simulink model "sampleModel1873_5_sub_sub"  (R2023a)
settings: Solver=VariableStepAuto  StartTime=0.0  StopTime=10.0  RelTol=1e-3
libraries: hdlsllib x7, simulink x1
settings Model: Creator=user1  LastModifiedBy=user1

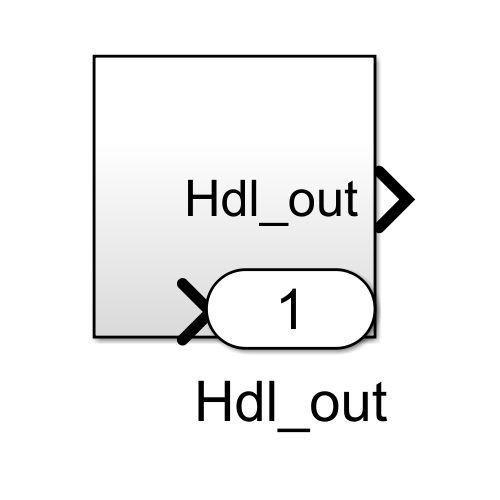
[thumbnail: Simulink's stored preview of the top-level diagram]
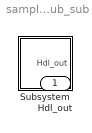
== system sampleModel1873_5_sub_sub ==
  Subsystem : Subsystem
  Hdl_out : Outport  OutDataTypeStr=uint8

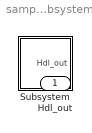
== system sampleModel1873_5_sub_sub/Subsystem ==
  Subsystem : Subsystem
  Hdl_out : Outport  OutDataTypeStr=uint8

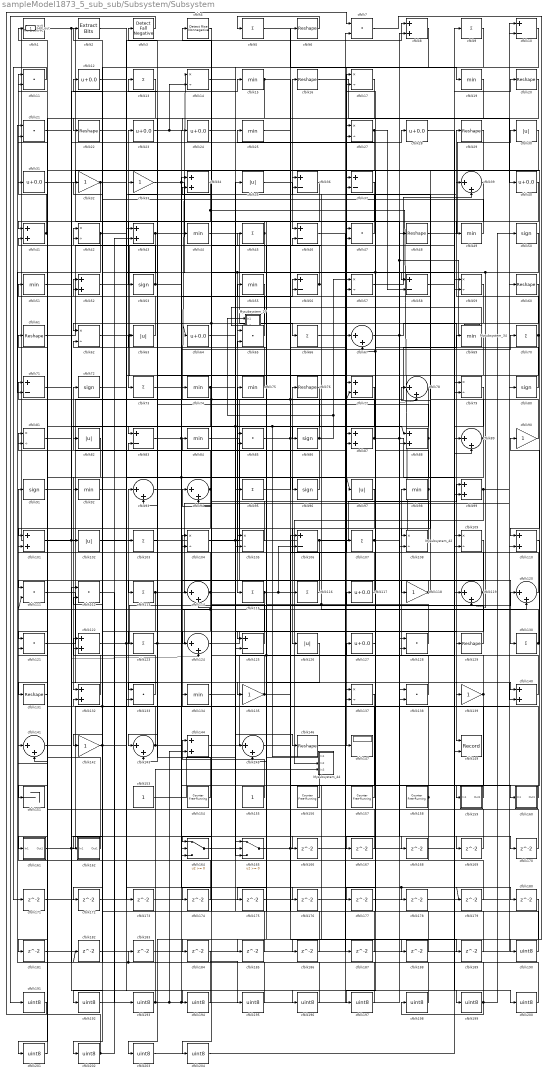
== system sampleModel1873_5_sub_sub/Subsystem/Subsystem ==
  Mysubsystem_27 : Subsystem  TreatAsAtomicUnit=on  RTWFcnName=Mysubsystem_27
      settings: RTWFcnNameOpts=User specified  RTWFileNameOpts=Use function name
  Mysubsystem_34 : Subsystem  TreatAsAtomicUnit=on  RTWFcnName=Mysubsystem_34
      settings: RTWFcnNameOpts=User specified  RTWFileNameOpts=Use function name
  Mysubsystem_42 : Subsystem  TreatAsAtomicUnit=on  RTWFcnName=Mysubsystem_42
      settings: RTWFcnNameOpts=User specified  RTWFileNameOpts=Use function name
  Mysubsystem_44 : Subsystem  TreatAsAtomicUnit=on  RTWFcnName=Mysubsystem_44
      settings: RTWFcnNameOpts=User specified  RTWFileNameOpts=Use function name
  cfblk1 : hdlsllib/Logic and Bit Operations/Detect Fall Nonpositive  vinit=0  OutDataTypeStr=uint8
  cfblk{10,36..37,46,56,58,71,83,106,125} (10 alike) : Sum  Inputs=+-  OutDataTypeStr=uint8
  cfblk{8,34,41,43,52,77,87..88,99,101,110,122,132,140,144} (15 alike) : Sum  OutDataTypeStr=uint8
  cfblk{30,35,63,82,97,102,126} (7 alike) : Abs  OutDataTypeStr=uint8  SaturateOnIntegerOverflow=off
  cfblk{5,9,13,45,66,70,73,95,103,107,113,115..116,123,130} (15 alike) : Sum  Inputs=+  OutDataTypeStr=uint8
  cfblk{14,17,27,42,57,59,62,79,81,104..105,108..109,137} (14 alike) : Product  Inputs=*/  OutDataTypeStr=uint8  RndMeth=Zero  SaturateOnIntegerOverflow=on
  cfblk{7,11,21,47,65,85,111..112,121,128,133,138} (12 alike) : DotProduct  OutDataTypeStr=uint8
  cfblk{39,67,78,89,93..94,114,119..120,124,141,143,145} (13 alike) : Sum  Inputs=|++  OutDataTypeStr=uint8
  cfblk{12,23..24,28,31,40,64,117,127} (9 alike) : Bias  Bias=0.0  SaturateOnIntegerOverflow=off
  cfblk{32..33,90,118,135,139,142} (7 alike) : Gain  OutDataTypeStr=uint8
  cfblk{6,16,20,22,29,48,60..61,76,129,131,146} (12 alike) : Reshape
  cfblk{15,19,25,44,49,51,55,69,74..75,84,92,98,134} (14 alike) : MinMax  OutDataTypeStr=uint8
  cfblk147 : Display
  cfblk149 : Record  FileSettingsInternal="{\"entries\":[{\"content\":{\"excelSettings\":{\"content\":{},\"type\":\"Streamout.ExcelSettings\"}},\"type\":\"Streamout.FileSettingStorage\",\"uuid\":\"\"}],\"packageUris\":[\"http:\\/\\/schema.mathworks.com\\/mf0\\/streamout_blocks\\/R2020a\"],\"version\":\"1.0\"}"  Layout=[1 1]  SignalsInternal="{\"entries\":[{\"content\":{\"signals\":[{\"content\":{\"blockPath\":[],\"dimensions\":[1],\"domain\":\"\",\"lineColor\":\"#a2142f\",\"plots\":[1],\"port\":1,\"signalID\":46057,\"signalName\":\"cfblk67\"},\"type\":\"RecordBlkView.Signal\",\"uuid\":\"\"},{\"content\":{\"blockPath\":[],\"dimensions\":[1],\"domain\":\"\",\"lineColor\":\"#139fff\",\"plots\":[1],\"port\":2,\"signalID\":46060,\"signalName\":\"cfblk87\"},\"type\":\"RecordBlkView.Signal\",\"uuid\":\"\"}]},\"type\":\"RecordBlkView.InputSignals\",\"uuid\":\"\"}],\"packageUris\":[\"http:\\/\\/schema.mathworks.com\\/mf0\\/streamout_blocks\\/R2020a\"],\"version\":\"1.0\"}"  VisualizationBindings="{\"xyplotplugin\":{\"info\":[{\"series\":[{\"bindingParametersList\":[{\"parameter\":\"X-Axis\",\"signalID\":46057,\"signalName\":\"cfblk67\"},{\"parameter\":\"Y-Axis\",\"signalID\":46060,\"signalName\":\"cfblk87\"}],\"seriesID\":10665}],\"subplotID\":1}]}}"  CompatibilityTag=XY  st=-1
  cfblk151 : Terminator
  cfblk153 : Constant  OutDataTypeStr=uint8  SampleTime=-1
  cfblk{154,156..158} (4 alike) : hdlsllib/Sources/Counter Free-Running  NumBits=16  tsamp=-1
  cfblk155 : Constant  OutDataTypeStr=uint8  SampleTime=-1
  cfblk159 : Subsystem
      settings: LibrarySourceBlock=|
      | hdlsllib/Ports &
      | Subsystems/Subsystem
  cfblk160 : Subsystem
      settings: LibrarySourceBlock=|
      | hdlsllib/Ports &
      | Subsystems/Subsystem
  cfblk161 : Subsystem
      settings: LibrarySourceBlock=|
      | hdlsllib/Ports &
      | Subsystems/Subsystem
  cfblk162 : Subsystem
      settings: LibrarySourceBlock=|
      | hdlsllib/Ports &
      | Subsystems/Subsystem
  cfblk164 : Switch  OutDataTypeStr=uint8  SaturateOnIntegerOverflow=off  InputSameDT=off
  cfblk165 : Switch  OutDataTypeStr=uint8  SaturateOnIntegerOverflow=off  InputSameDT=off
  cfblk{166..189} (24 alike) : Delay  SampleTime=1
  cfblk{190..204} (15 alike) : DataTypeConversion  OutDataTypeStr=uint8  SaturateOnIntegerOverflow=off  RndMeth=Floor
  cfblk2 : simulink/Logic and Bit Operations/Extract Bits  bitsToExtract=Upper half  numBits=8  bitIdxRange=[0 7]  outScalingMode=Preserve fixed-point scaling
      settings: LibrarySourceBlock=|
      | hdlsllib/Logic and Bit
      | Operations/Extract Bits
  cfblk3 : hdlsllib/Logic and Bit Operations/Detect Fall Negative  vinit=0  OutDataTypeStr=uint8
  cfblk4 : hdlsllib/Logic and Bit Operations/Detect Rise Nonnegative  vinit=0  OutDataTypeStr=uint8
  cfblk{50,53,72,80,86,91,96} (7 alike) : Signum
  Hdl_out : Outport  OutDataTypeStr=uint8
  wires:
  Mysubsystem_34/1(Out1) -> Mysubsystem_27/2(In2)
  cfblk204/1 -> cfblk59/2
  cfblk203/1 -> cfblk59/1
  cfblk180/1 -> cfblk203/1
  cfblk202/1 -> cfblk121/2, cfblk43/2
  cfblk201/1 -> cfblk141/2
  cfblk200/1 -> cfblk141/1
  cfblk28/1 -> cfblk200/1
  cfblk199/1 -> cfblk183/1, cfblk182/1, cfblk198/1, cfblk50/1
  cfblk198/1 -> cfblk21/2
  cfblk197/1 -> cfblk21/1
  cfblk196/1 -> cfblk34/1
  cfblk21/1 -> cfblk196/1
  cfblk195/1 -> cfblk112/2
  cfblk184/1 -> cfblk195/1
  cfblk194/1 -> cfblk112/1
  cfblk12/1 -> cfblk194/1
  cfblk193/1 -> Mysubsystem_44/3(In3), cfblk48/1, Mysubsystem_34/1(In1), cfblk44/1, cfblk144/2
  cfblk192/1 -> cfblk7/2
  cfblk191/1 -> cfblk7/1
  cfblk3/1 -> cfblk191/1
  cfblk190/1 -> cfblk165/1
  cfblk7/1 -> cfblk190/1
  cfblk189/1 -> cfblk17/2
  cfblk25/1 -> cfblk189/1
  cfblk188/1 -> cfblk106/1
  cfblk187/1 -> cfblk94/1
  cfblk66/1 -> cfblk187/1
  cfblk186/1 -> cfblk65/2
  cfblk137/1 -> cfblk186/1
  cfblk185/1 -> cfblk132/2
  cfblk36/1 -> cfblk185/1
  cfblk4/1 -> cfblk184/1
  cfblk183/1 -> cfblk138/2
  cfblk182/1 -> cfblk10/2
  cfblk181/1 -> cfblk114/1
  cfblk77/1 -> cfblk181/1
  cfblk145/1 -> cfblk180/1
  cfblk179/1 -> cfblk85/2
  cfblk178/1 -> cfblk99/2
  cfblk177/1 -> cfblk89/2
  cfblk29/1 -> cfblk177/1
  cfblk176/1 -> cfblk88/2
  cfblk175/1 -> cfblk110/2
  cfblk126/1 -> cfblk175/1
  cfblk174/1 -> cfblk81/2
  cfblk173/1 -> cfblk109/1
  cfblk72/1 -> cfblk173/1
  cfblk172/1 -> cfblk43/1
  cfblk171/1 -> cfblk105/2
  cfblk11/1 -> cfblk171/1
  cfblk170/1 -> cfblk122/2
  cfblk169/1 -> cfblk62/2
  cfblk168/1 -> cfblk79/1
  cfblk167/1 -> cfblk1/1
  cfblk127/1 -> cfblk167/1
  cfblk166/1 -> cfblk128/1
  cfblk73/1 -> cfblk166/1
  cfblk50/1 -> cfblk64/1, cfblk174/1, cfblk197/1, cfblk119/2
  cfblk132/1 -> cfblk122/1
  cfblk125/1 -> cfblk81/1
  cfblk19/1 -> cfblk123/1
  cfblk159/1(Out1) -> cfblk114/2
  cfblk134/1 -> cfblk120/1
  cfblk114/1 -> cfblk111/2, cfblk192/1, cfblk47/1, cfblk63/1
  cfblk62/1 -> cfblk116/1, cfblk9/1
  cfblk115/1 -> cfblk107/1, cfblk106/2, cfblk164/2
  cfblk122/1 -> cfblk117/1, cfblk36/2
  cfblk35/1 -> cfblk46/1
  cfblk83/1 -> cfblk56/1, cfblk137/2
  cfblk90/1 -> cfblk55/1
  cfblk107/1 -> cfblk8/2, Hdl_out/1
  cfblk51/1 -> cfblk135/1
  cfblk165/1 -> cfblk119/1, cfblk188/1
  cfblk33/1 -> cfblk134/1, cfblk145/1
  cfblk30/1 -> cfblk108/1
  cfblk144/1 -> cfblk89/1
  cfblk56/1 -> cfblk4/1, cfblk36/1
  cfblk14/1 -> cfblk88/1, cfblk169/1
  cfblk24/1 -> cfblk128/2
  cfblk13/1 -> cfblk162/1(In1)
  cfblk74/1 -> cfblk143/2, cfblk146/1
  cfblk109/1 -> cfblk161/1(In1)
  cfblk22/1 -> cfblk58/1
  cfblk49/1 -> cfblk12/1
  cfblk128/1 -> cfblk45/1, cfblk56/2
  cfblk15/1 -> cfblk37/1, cfblk201/1
  cfblk102/1 -> cfblk8/1
  cfblk23/1 -> cfblk118/1, cfblk14/2
  cfblk97/1 -> cfblk126/1
  cfblk57/1 -> cfblk39/2
  cfblk112/1 -> cfblk193/1
  cfblk27/1 -> cfblk121/1, cfblk58/2
  cfblk9/1 -> cfblk125/2
  cfblk130/1 -> cfblk90/1, cfblk46/2
  cfblk58/1 -> cfblk20/1
  cfblk2/1 -> cfblk178/1, cfblk179/1
  cfblk20/1 -> cfblk24/1
  cfblk153/1 -> cfblk35/1
  cfblk79/1 -> cfblk109/2
  cfblk95/1 -> cfblk77/2, cfblk67/1
  cfblk53/1 -> cfblk97/1, cfblk176/1, cfblk11/2
  cfblk76/1 -> cfblk204/1, Mysubsystem_44/1(In1)
  cfblk16/1 -> cfblk40/1
  cfblk43/1 -> cfblk102/1, cfblk79/2
  cfblk81/1 -> cfblk15/1
  cfblk106/1 -> cfblk99/1, cfblk133/2
  cfblk80/1 -> cfblk25/1
  cfblk75/1 -> cfblk52/2
  cfblk138/1 -> cfblk105/1, cfblk74/1
  cfblk103/1 -> cfblk143/1
  cfblk42/1 -> cfblk77/1, cfblk71/2
  cfblk59/1 -> cfblk202/1
  cfblk91/1 -> cfblk27/2
  cfblk34/1 -> Mysubsystem_42/1(In1), cfblk53/1
  cfblk139/1 -> cfblk85/1, cfblk164/3
  cfblk5/1 -> cfblk19/1
  cfblk86/1 -> Mysubsystem_27/1(In1), cfblk57/1, cfblk14/1, cfblk34/2
  cfblk89/1 -> cfblk125/1, cfblk37/2
  cfblk111/1 -> cfblk139/1
  cfblk146/1 -> cfblk39/1
  cfblk108/1 -> cfblk83/2
  cfblk131/1 -> cfblk71/1
  cfblk129/1 -> cfblk104/2
  cfblk17/1 -> cfblk22/1
  cfblk87/1 -> cfblk149/2, cfblk170/1, cfblk41/2
  cfblk93/1 -> cfblk70/1
  cfblk164/1 -> cfblk127/1
  cfblk162/1(Out1) -> cfblk31/1
  cfblk141/1 -> cfblk199/1
  cfblk60/1 -> cfblk94/2
  cfblk65/1 -> cfblk13/1
  cfblk133/1 -> cfblk2/1
  cfblk69/1 -> cfblk83/1
  cfblk46/1 -> cfblk87/2
  cfblk155/1 -> cfblk144/1
  cfblk119/1 -> cfblk93/2, cfblk145/2
  cfblk37/1 -> cfblk92/1
  cfblk101/1 -> cfblk87/1, cfblk28/1, cfblk165/3
  cfblk94/1 -> cfblk32/1, cfblk131/1
  cfblk1/1 -> cfblk138/1, cfblk137/1
  cfblk64/1 -> cfblk95/1
  cfblk39/1 -> cfblk49/1
  cfblk98/1 -> cfblk57/2, cfblk67/2, cfblk172/1
  cfblk52/1 -> cfblk23/1
  cfblk156/1 -> cfblk101/2
  cfblk160/1(Out1) -> cfblk104/1
  cfblk44/1 -> cfblk66/1
  cfblk104/1 -> cfblk69/1, cfblk140/2
  cfblk85/1 -> cfblk140/1, cfblk47/2
  cfblk113/1 -> cfblk80/1, cfblk142/1
  cfblk41/1 -> cfblk11/1, cfblk111/1
  cfblk99/1 -> Mysubsystem_44/2(In2), cfblk10/1
  cfblk78/1 -> cfblk164/1
  cfblk84/1 -> cfblk130/1
  cfblk157/1 -> cfblk61/1, cfblk42/2
  cfblk161/1(Out1) -> cfblk60/1, cfblk124/2
  cfblk154/1 -> cfblk52/1
  cfblk105/1 -> cfblk82/1
  cfblk10/1 -> cfblk62/1
  cfblk48/1 -> cfblk30/1
  cfblk71/1 -> cfblk86/1
  cfblk61/1 -> cfblk27/1
  cfblk120/1 -> cfblk75/1
  cfblk110/1 -> cfblk159/1(In1)
  cfblk135/1 -> cfblk84/1, cfblk160/1(In1)
  cfblk140/1 -> cfblk98/1
  cfblk45/1 -> cfblk65/1, cfblk124/1, cfblk41/1
  cfblk70/1 -> cfblk29/1, cfblk133/1
  cfblk32/1 -> cfblk151/1, cfblk168/1
  cfblk121/1 -> cfblk6/1
  cfblk124/1 -> cfblk129/1
  cfblk63/1 -> cfblk51/1
  cfblk55/1 -> cfblk115/1
  cfblk88/1 -> cfblk101/1, cfblk3/1
  cfblk117/1 -> cfblk17/1
  cfblk123/1 -> cfblk103/1, cfblk108/2
  cfblk92/1 -> cfblk96/1
  cfblk47/1 -> cfblk16/1
  cfblk6/1 -> cfblk5/1
  cfblk8/1 -> cfblk147/1
  cfblk96/1 -> cfblk72/1
  cfblk142/1 -> cfblk42/1, cfblk165/2
  cfblk82/1 -> cfblk132/1
  cfblk158/1 -> cfblk91/1, cfblk33/1
  cfblk31/1 -> cfblk110/1
  cfblk67/1 -> cfblk149/1, cfblk78/2
  cfblk116/1 -> cfblk76/1
  cfblk118/1 -> cfblk113/1, cfblk78/1
  cfblk143/1 -> cfblk93/1, cfblk120/2
  cfblk40/1 -> cfblk73/1

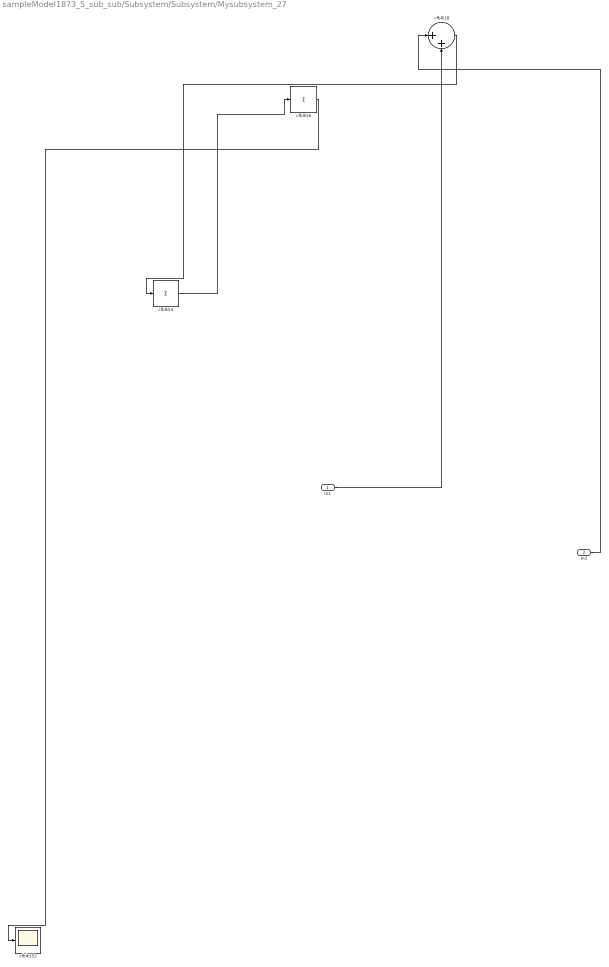
== system sampleModel1873_5_sub_sub/Subsystem/Subsystem/Mysubsystem_27 ==
  In1 : Inport
  In2 : Inport  Port=2
  cfblk152 : Scope
  cfblk18 : Sum  Inputs=|++
  cfblk26 : Sum  Inputs=+
  cfblk54 : Sum  Inputs=+
  wires:
  cfblk54/1 -> cfblk26/1
  cfblk18/1 -> cfblk54/1
  In2/1 -> cfblk18/1
  cfblk26/1 -> cfblk152/1
  In1/1 -> cfblk18/2

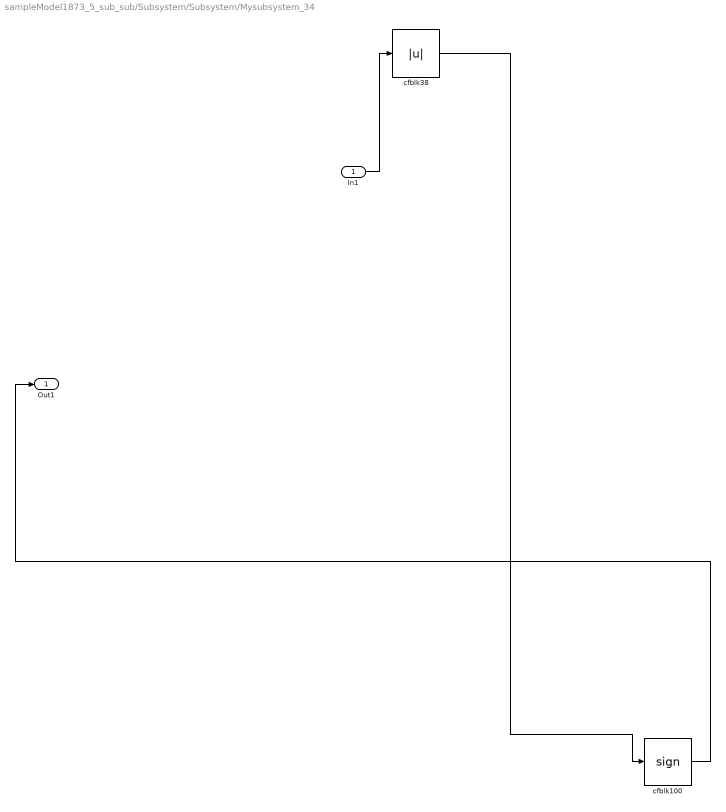
== system sampleModel1873_5_sub_sub/Subsystem/Subsystem/Mysubsystem_34 ==
  In1 : Inport
  cfblk100 : Signum
  cfblk38 : Abs  SaturateOnIntegerOverflow=off
  Out1 : Outport
  wires:
  In1/1 -> cfblk38/1
  cfblk38/1 -> cfblk100/1
  cfblk100/1 -> Out1/1

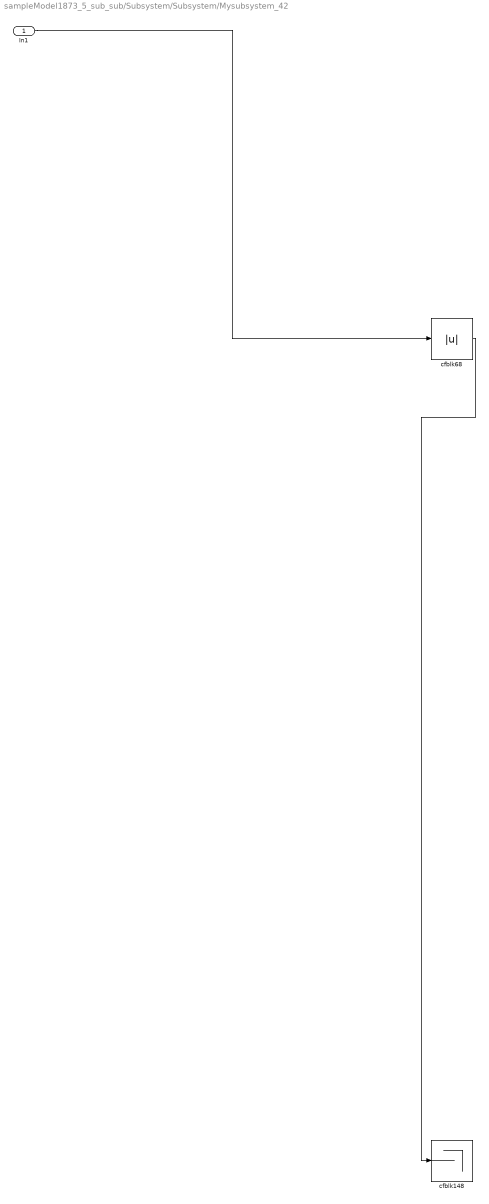
== system sampleModel1873_5_sub_sub/Subsystem/Subsystem/Mysubsystem_42 ==
  In1 : Inport
  cfblk148 : Terminator
  cfblk68 : Abs  SaturateOnIntegerOverflow=off
  wires:
  In1/1 -> cfblk68/1
  cfblk68/1 -> cfblk148/1

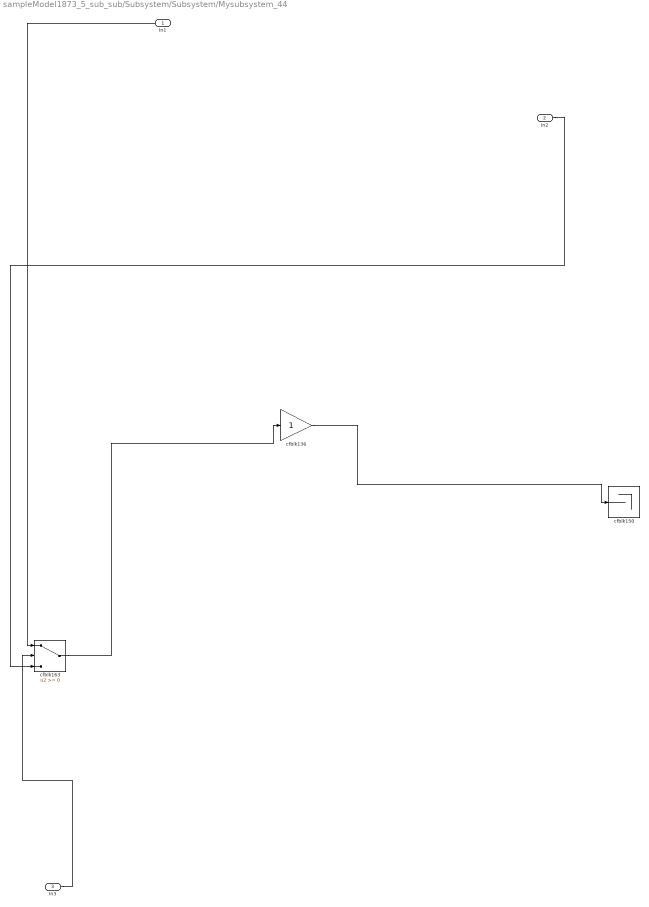
== system sampleModel1873_5_sub_sub/Subsystem/Subsystem/Mysubsystem_44 ==
  In1 : Inport
  In2 : Inport  Port=2
  In3 : Inport  Port=3
  cfblk136 : Gain
  cfblk150 : Terminator
  cfblk163 : Switch  SaturateOnIntegerOverflow=off  InputSameDT=off
  wires:
  cfblk163/1 -> cfblk136/1
  In2/1 -> cfblk163/3
  cfblk136/1 -> cfblk150/1
  In3/1 -> cfblk163/2
  In1/1 -> cfblk163/1

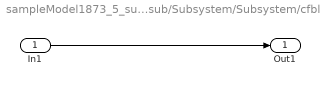
== system sampleModel1873_5_sub_sub/Subsystem/Subsystem/cfblk159 ==
  In1 : Inport
  Out1 : Outport
  wires:
  In1/1 -> Out1/1

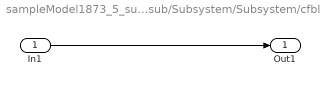
== system sampleModel1873_5_sub_sub/Subsystem/Subsystem/cfblk160 ==
  In1 : Inport
  Out1 : Outport
  wires:
  In1/1 -> Out1/1

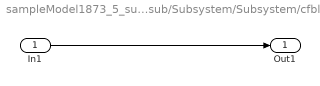
== system sampleModel1873_5_sub_sub/Subsystem/Subsystem/cfblk161 ==
  In1 : Inport
  Out1 : Outport
  wires:
  In1/1 -> Out1/1

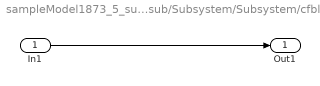
== system sampleModel1873_5_sub_sub/Subsystem/Subsystem/cfblk162 ==
  In1 : Inport
  Out1 : Outport
  wires:
  In1/1 -> Out1/1
